simulink model "YTT"  (R2020b)
settings: Solver=VariableStepAuto  StartTime=0.0  StopTime=150  RelTol=1e-3
libraries: simulink x1, mpclib x1
settings Model: Creator=LJD  LastModifiedBy=LJD

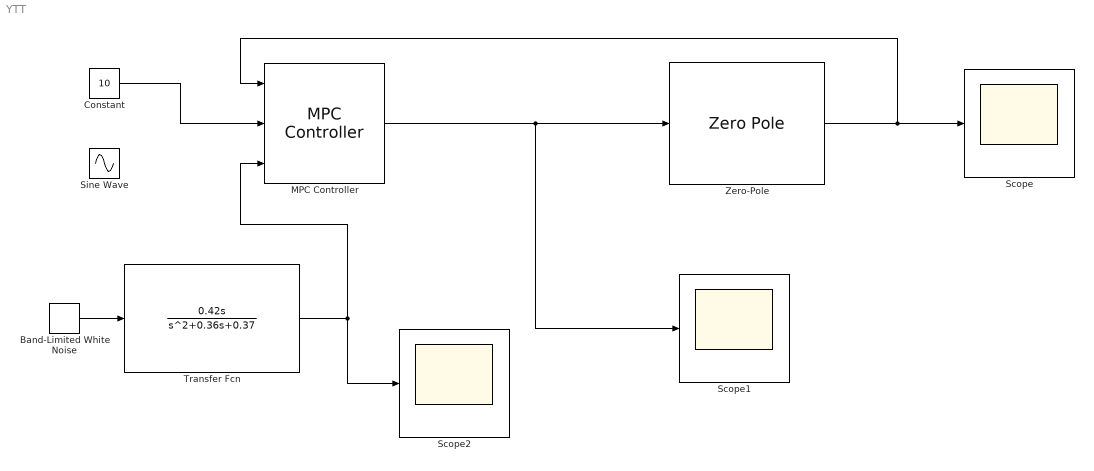
== system YTT ==
  Band-Limited White Noise : simulink/Sources/Band-Limited White Noise  Cov=[0.1]  Ts=0.1  seed=[23341]
  Constant : Constant  Value=10
  MPC Controller : mpclib/MPC Controller  SCDEnableBlockLinearizationSpecification=on  mpcobj=mpc1  is_multiple=0  enable_value=0  return_u0=off  updateMPCinCallerWorkspace=on  md_inport=on  mv_inport=off  uref_inport=off  return_cost=off  return_mvseq=off  return_qpstatus=off  return_xseq=off  return_state=off  return_ovseq=off  state_inport=off  umin_inport=off  umax_inport=off  ymin_inport=off  ymax_inport=off  cc_inport=off  ywt_inport=off  uwt_inport=off  duwt_inport=off  rhoeps_inport=off  pm_inport=off  MaximumP=10  HorizonChoice=FixedHorizon  n_ts=0.1  n_p=10  n_mv=1  n_md=1  n_ud=0  n_mo=1  n_uo=0  BlockDataType=double  SampleTimeInherited=off  switch_inport=off
  Scope : Scope
  Scope1 : Scope
  Scope2 : Scope
  Sine Wave : Sin  Amplitude=90  Frequency=0.02  SampleTime=0
  Transfer Fcn : TransferFcn  Numerator=[0.42 0]  Denominator=[1 0.36 0.37]
  Zero-Pole : ZeroPole  Zeros=[]  Poles=[0 -0.52]  Gain=0.25
  wires:
  MPC Controller/1 -> Scope1/1, Zero-Pole/1
  Zero-Pole/1 -> MPC Controller/1, Scope/1
  Transfer Fcn/1 -> MPC Controller/3, Scope2/1
  Constant/1 -> MPC Controller/2
  Band-Limited White Noise/1 -> Transfer Fcn/1
